simulink model "trajectory_ctrl_unicycle"  (R2021b)
settings: Solver=FixedStepAuto  StartTime=0.0  StopTime=T  FixedStep=Ts  RelTol=1e-3
values from neighbouring files (symbols this model uses):
  k1 = 2*csi*a    (= 8)    [def_trajectory.m]    (also in def_trajectory_smagrito_fixato.m = 35)
  k2 = (a^2 - w_des^2)/(v_des)    (= 152.782200384)    [def_trajectory.m]    (also in def_trajectory_smagrito_fixato.m = 1200)
  k3 = k1    (= 8)    [def_trajectory.m]    (also in def_trajectory_smagrito_fixato.m = 35)
  rect_samples = ceil(theta_samples / (2*pi))    [def_trajectory.m]    (also in def_trajectory_smagrito_fixato.m)
  Ts = 0.01    [def_trajectory.m]
  v_des = (2*pi*r0)/(T)    (= 0.418879020479)    [def_trajectory.m]    (also in def_trajectory_smagrito_fixato.m = 1)
  w_des = (2*pi)/T    (= 0.0523598775598)    [def_trajectory.m]    (also in def_trajectory_smagrito_fixato.m = 5)
undefined symbols (not defined in the file or in its folder): unicycle
settings Model: Creator=Riccardo Barbiero  LastModifiedBy=Riccardo Barbiero

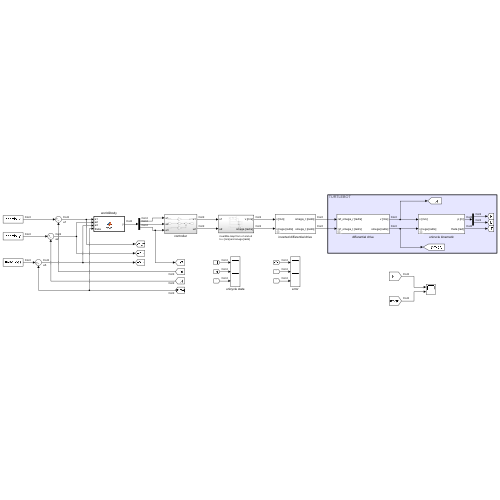
[thumbnail: Simulink's stored preview of the top-level diagram]
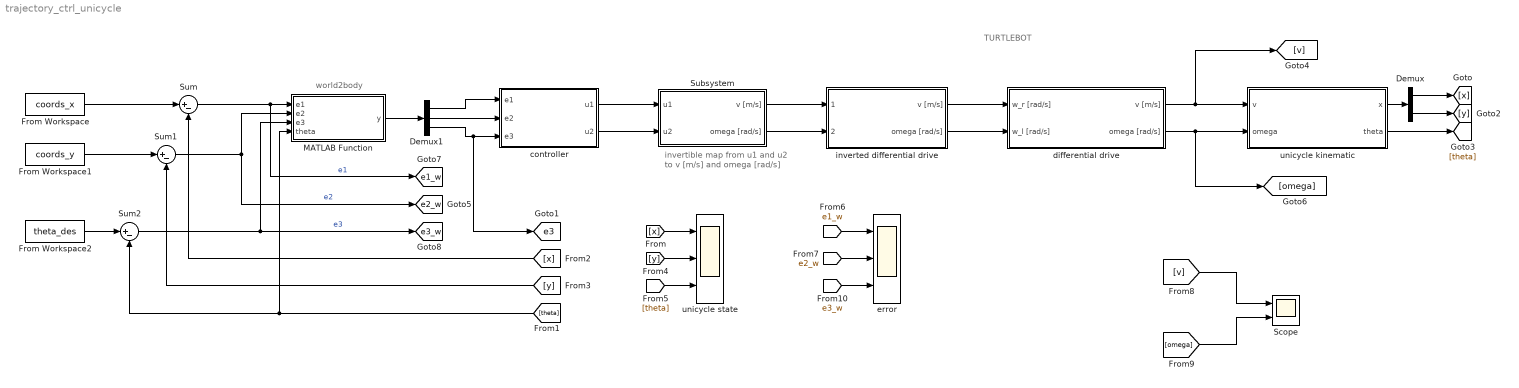
== system trajectory_ctrl_unicycle ==
  note: world2body
  note: invertible map from u1 and u2
      | to v [m/s] and omega [rad/s]
  note: TURTLEBOT
  Demux : Demux  Outputs=2
  Demux1 : Demux  Outputs=3
  From Workspace : FromWorkspace  VariableName=coords_x
  From Workspace1 : FromWorkspace  VariableName=coords_y
  From Workspace2 : FromWorkspace  VariableName=theta_des
  MATLAB Function : MATLAB Function  TreatAsAtomicUnit=on
  Scope : Scope  NumInputPorts=2
  Subsystem : Subsystem
  Sum : Sum  Inputs=|+-
  Sum1 : Sum  Inputs=|+-
  Sum2 : Sum  Inputs=|+-
  controller : Subsystem
  differential drive : Subsystem  mask(Differential drive for a unicycle){r=unicycle.diffDrive.r, d=unicycle.diffDrive.d, wheelDyEn=on, Tc=unicycle.diffDrive.Td, wheelsSpeedUpperLimit=unicycle.diffDrive.omegaWheelMax, wheelsSpeedLowerLimit=unicycle.diffDrive.omegaWheelMin}
      mask prompts: r "wheel radius"; d "interaxis lenght"; wheelDyEn "l.p.f. enable"; Tc "time constant [s]"; wheelsSpeedUpperLimit "max wheel speed  [rad/s]"; wheelsSpeedLowerLimit "min wheel speed [rad/s]"
      mask help:
      | Model of a differential drive.
      | It takes as input the derired wheel velocities and converts them to the corresponding driving velocity and stearing velocity.
      | Wheels dynamics can be taken into accont, along with output saturation.
      mask Help:
      | author: Beniamino Pozzan
      | email: beniamino.pozzan@phd.unipd.it
      mask Callback wheelDyEn:
      | % get the enable parameter
      | wheelDyEnStatus = get_param(gcb,'wheelDyEn');
      | enableStatus = get_param(gcb,'MaskEnables');
      | % if it is true, make Tc enabled
      | if strcmp(wheelDyEnStatus,'on')
      |     enableStatus{4}='on';
      | else
      |     enableStatus{4}='off';
      | end
      | set_param(gcb,'MaskEnables',enableStatus)
      mask TypeOptions wheelsSpeedUpperLimit: w_l saturator/UpperLimit | w_r saturator/UpperLimit
      mask TypeOptions wheelsSpeedLowerLimit: w_l saturator/LowerLimit | w_r saturator/LowerLimit
      mask DialogControl wheelDy Prompt: wheel dynamics
  error : Scope  NumInputPorts=3
  inverted differential drive : Subsystem  mask(Inverted Differential drive for a unicycle){r=unicycle.diffDrive.r, d=unicycle.diffDrive.d}
      mask prompts: r "wheel radius"; d "interaxis lenght"
      mask help:
      | Inverted differential drive for a unicycle.
      | Provided the desired driving and stearing velocities, it computes the corresponding wheel velocities.
  unicycle kinematic : Subsystem  mask(Unicycle Kinematic Model){x0=unicycle.ic.x, y0=unicycle.ic.y, theta0=unicycle.ic.theta}
      mask prompts: x0 "x_0"; y0 "y_0"; theta0 "theta_0"
      mask help: kinematic model of a unicyle.
  unicycle state : Scope  NumInputPorts=3
  tag scope: e1_w=global, e2_w=global, e3=global, e3_w=global
  wires:
  differential drive/1(v [m/s]) -> [v], unicycle kinematic/1(v)
  inverted differential drive/2(omega [rad/s]) -> differential drive/2(w_l [rad/s])
  differential drive/2(omega [rad/s]) -> [omega], unicycle kinematic/2(omega)
  inverted differential drive/1(v [m/s]) -> differential drive/1(w_r [rad/s])
  Sum2/1 -> MATLAB Function/3(e3), [e3_w]  "e3"
  controller/1(u1) -> Subsystem/1(u1)
  controller/2(u2) -> Subsystem/2(u2)
  Subsystem/1(v [m/s]) -> inverted differential drive/1(1)
  Subsystem/2(omega [rad/s]) -> inverted differential drive/2(2)
  From Workspace/1 -> Sum/1
  [x] -> Sum/2
  From Workspace1/1 -> Sum1/1
  [y] -> Sum1/2
  From Workspace2/1 -> Sum2/1
  [theta] -> Sum2/2, MATLAB Function/4(theta)
  Sum/1 -> MATLAB Function/1(e1), [e1_w]  "e1"
  Sum1/1 -> [e2_w], MATLAB Function/2(e2)  "e2"
  MATLAB Function/1(y) -> Demux1/1
  Demux1/2 -> controller/2(e2)
  Demux1/1 -> controller/1(e1)
  Demux1/3 -> controller/3(e3), [e3]
  [x] -> unicycle state/1
  [theta] -> unicycle state/3
  [y] -> unicycle state/2
  unicycle kinematic/1(x) -> Demux/1
  Demux/2 -> [y]
  Demux/1 -> [x]
  unicycle kinematic/2(theta) -> [theta]
  [e2_w] -> error/2
  [e3_w] -> error/3
  [e1_w] -> error/1
  [v] -> Scope/1
  [omega] -> Scope/2

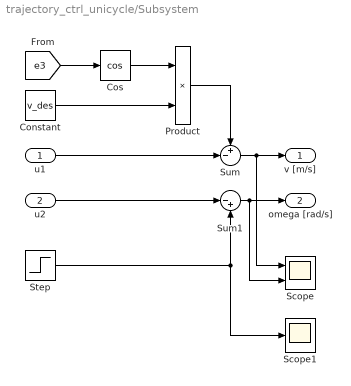
== system trajectory_ctrl_unicycle/Subsystem ==
  u1 : Inport
  u2 : Inport  Port=2
  Constant : Constant  Value=v_des
  Cos : Trigonometry  Operator=cos
  Product : Product
  Scope : Scope  NumInputPorts=2
  Scope1 : Scope
  Step : Step  Time=rect_samples*Ts  After=w_des  SampleTime=0
  Sum : Sum  Inputs=+-|
  Sum1 : Sum  Inputs=|-+
  v [m/s] : Outport
  omega [rad/s] : Outport  Port=2
  wires:
  [e3] -> Cos/1
  Constant/1 -> Product/2
  Cos/1 -> Product/1
  Sum/1 -> Scope/1, v [m/s]/1
  u1/1 -> Sum/2
  Product/1 -> Sum/1
  u2/1 -> Sum1/1
  Step/1 -> Scope1/1, Sum1/2
  Sum1/1 -> omega [rad/s]/1, Scope/2

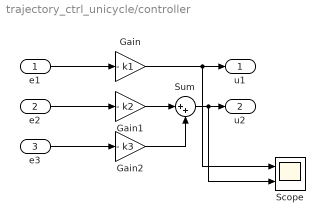
== system trajectory_ctrl_unicycle/controller ==
  e1 : Inport
  e2 : Inport  Port=2
  e3 : Inport  Port=3
  Gain : Gain  Gain=- k1
  Gain1 : Gain  Gain=- k2
  Gain2 : Gain  Gain=- k3
  Scope : Scope  NumInputPorts=2
  Sum : Sum  Inputs=|++
  u1 : Outport
  u2 : Outport  Port=2
  wires:
  e1/1 -> Gain/1
  Gain/1 -> Scope/1, u1/1
  e3/1 -> Gain2/1
  e2/1 -> Gain1/1
  Gain1/1 -> Sum/1
  Gain2/1 -> Sum/2
  Sum/1 -> Scope/2, u2/1

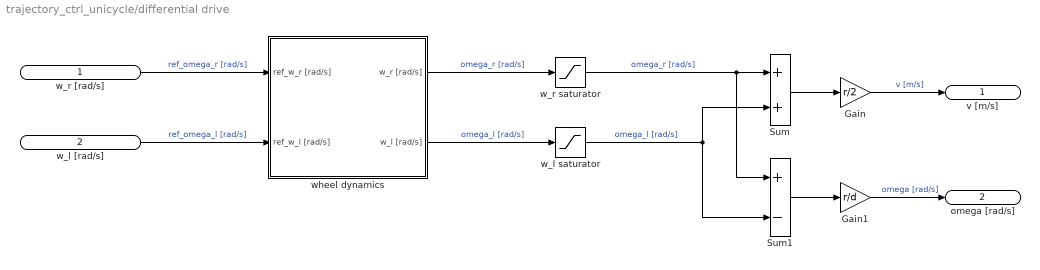
== system trajectory_ctrl_unicycle/differential drive ==
  w_r [rad/s] : Inport  Unit=rad/s
  w_l [rad/s] : Inport  Port=2  Unit=rad/s
  Gain : Gain  Gain=r/2
  Gain1 : Gain  Gain=r/d
  Sum : Sum
  Sum1 : Sum  Inputs=+-
  w_l saturator : Saturate  UpperLimit=wheelsSpeedUpperLimit  LowerLimit=wheelsSpeedLowerLimit
  w_r saturator : Saturate  UpperLimit=wheelsSpeedUpperLimit  LowerLimit=wheelsSpeedLowerLimit
  wheel dynamics : Subsystem  Variant=on
  v [m/s] : Outport  Unit=m/s
  omega [rad/s] : Outport  Port=2  Unit=rad/s
  wires:
  w_l saturator/1 -> Sum1/2, Sum/2  "omega_l [rad/s]"
  w_r saturator/1 -> Sum1/1, Sum/1  "omega_r [rad/s]"
  Gain1/1 -> omega [rad/s]/1  "omega [rad/s]"
  Sum1/1 -> Gain1/1
  Gain/1 -> v [m/s]/1  "v [m/s]"
  Sum/1 -> Gain/1
  w_r [rad/s]/1 -> wheel dynamics/1(ref_w_r [rad/s])  "ref_omega_r [rad/s]"
  w_l [rad/s]/1 -> wheel dynamics/2(ref_w_l [rad/s])  "ref_omega_l [rad/s]"
  wheel dynamics/1(w_r [rad/s]) -> w_r saturator/1  "omega_r [rad/s]"
  wheel dynamics/2(w_l [rad/s]) -> w_l saturator/1  "omega_l [rad/s]"

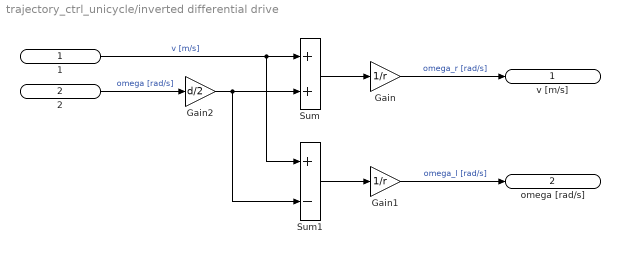
== system trajectory_ctrl_unicycle/inverted differential drive ==
  1 : Inport  Unit=m/s
  2 : Inport  Port=2  Unit=rad/s
  Gain : Gain  Gain=1/r
  Gain1 : Gain  Gain=1/r
  Gain2 : Gain  Gain=d/2
  Sum : Sum
  Sum1 : Sum  Inputs=+-
  v [m/s] : Outport  Unit=rad/s
  omega [rad/s] : Outport  Port=2  Unit=rad/s
  wires:
  Gain2/1 -> Sum1/2, Sum/2
  Sum/1 -> Gain/1
  Gain/1 -> v [m/s]/1  "omega_r [rad/s]"
  Sum1/1 -> Gain1/1
  Gain1/1 -> omega [rad/s]/1  "omega_l [rad/s]"
  1/1 -> Sum1/1, Sum/1  "v [m/s]"
  2/1 -> Gain2/1  "omega [rad/s]"

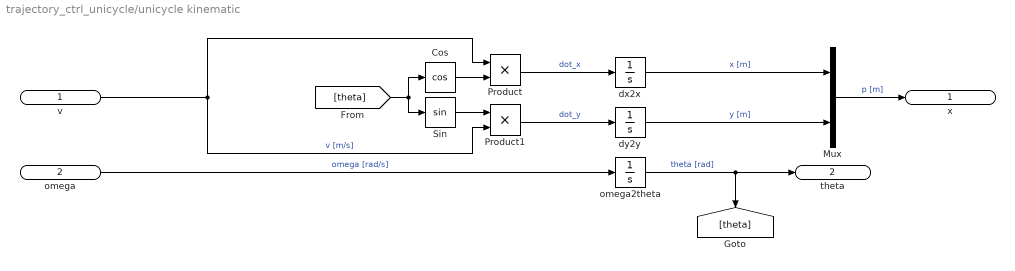
== system trajectory_ctrl_unicycle/unicycle kinematic ==
  v : Inport  PortDimensions=1
  omega : Inport  Port=2  PortDimensions=1
  Cos : Trigonometry  Operator=cos
  Mux : Mux  Inputs=2
  Product : Product
  Product1 : Product
  Sin : Trigonometry
  dx2x : Integrator  InitialCondition=x0  ContinuousStateAttributes='pos_x'
  dy2y : Integrator  InitialCondition=y0  ContinuousStateAttributes='pos_y'
  omega2theta : Integrator  InitialCondition=theta0  ContinuousStateAttributes='theta'
  x : Outport  PortDimensions=2
  theta : Outport  Port=2  PortDimensions=1
  wires:
  Product1/1 -> dy2y/1  "dot_y"
  [theta] -> Sin/1, Cos/1
  v/1 -> Product/1, Product1/2  "v [m/s]"
  omega2theta/1 -> [theta], theta/1  "theta [rad]"
  omega/1 -> omega2theta/1  "omega [rad/s]"
  dy2y/1 -> Mux/2  "y [m]"
  Cos/1 -> Product/2
  dx2x/1 -> Mux/1  "x [m]"
  Sin/1 -> Product1/1
  Product/1 -> dx2x/1  "dot_x"
  Mux/1 -> x/1  "p [m]"

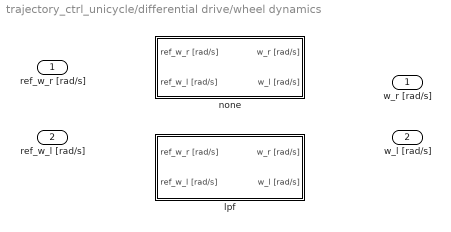
== system trajectory_ctrl_unicycle/differential drive/wheel dynamics ==
  ref_w_r [rad/s] : Inport
  ref_w_l [rad/s] : Inport  Port=2
  lpf : Subsystem  VariantControl=wheelDyEn==true
  none : Subsystem  VariantControl=wheelDyEn==false
  w_r [rad/s] : Outport
  w_l [rad/s] : Outport  Port=2

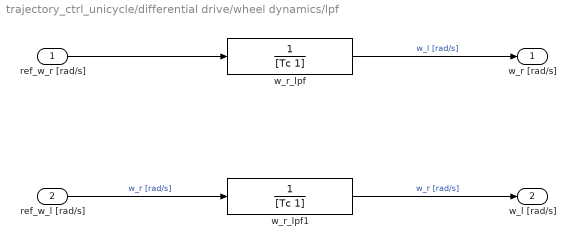
== system trajectory_ctrl_unicycle/differential drive/wheel dynamics/lpf ==
  ref_w_r [rad/s] : Inport
  ref_w_l [rad/s] : Inport  Port=2
  w_r_lpf : TransferFcn  Denominator=[Tc 1]  ContinuousStateAttributes='w_r_lpf'
  w_r_lpf1 : TransferFcn  Denominator=[Tc 1]  ContinuousStateAttributes='w_r_lpf'
  w_r [rad/s] : Outport
  w_l [rad/s] : Outport  Port=2
  wires:
  ref_w_r [rad/s]/1 -> w_r_lpf/1
  w_r_lpf1/1 -> w_l [rad/s]/1  "w_r [rad/s]"
  w_r_lpf/1 -> w_r [rad/s]/1  "w_l [rad/s]"
  ref_w_l [rad/s]/1 -> w_r_lpf1/1  "w_r [rad/s]"

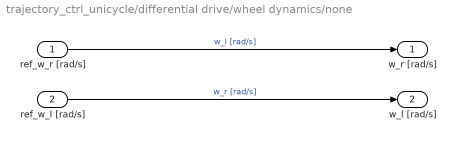
== system trajectory_ctrl_unicycle/differential drive/wheel dynamics/none ==
  ref_w_r [rad/s] : Inport
  ref_w_l [rad/s] : Inport  Port=2
  w_r [rad/s] : Outport
  w_l [rad/s] : Outport  Port=2
  wires:
  ref_w_r [rad/s]/1 -> w_r [rad/s]/1  "w_l [rad/s]"
  ref_w_l [rad/s]/1 -> w_l [rad/s]/1  "w_r [rad/s]"

== matlab function trajectory_ctrl_unicycle/MATLAB Function ==
  data: e1 input; y output; e2 input; e3 input; theta input
function y = w2b(e1, e2, e3, theta)
x = [e1;e2;e3]; 
mat = [cos(theta), -sin(theta), 0;
       sin(theta), cos(theta), 0;
       0, 0, 1];
u = ones(3,1);
u = mat'*x;
y = u;
